simulink library "controlLibrary"  (R2019b)
settings: Solver=VariableStepAuto  StartTime=0.0  StopTime=10.0  RelTol=1e-3
undefined symbols (not defined in the file or in its folder): DiscIntNeverNeededParam, Up
libraries: simulink x5
settings Model: Creator=mwalker  LastModifiedBy=agonzale

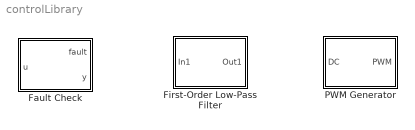
== system controlLibrary ==
  Fault Check : MATLAB Function  TreatAsAtomicUnit=on
  First-Order Low-Pass Filter : Subsystem  mask(First-Order Low-Pass Filter){fc=0.1}
      mask prompts: fc "Filter Constant"
      mask Display: disp(get_param(gcb,'fc'))
  PWM Generator : Subsystem  mask(PWM Generator){CarrCount=Up, Tper=0.001/0.05, Ts=0.001}
      mask prompts: CarrCount "Carrier counter:"; Tper "Timer period (s):"; Ts "Sample time"
      mask help:
      | This block implements a PWM generator.
      |
      | For discrete-time, set Sample time to a positive value. For continuous-time, set Sample time to zero.
      mask TypeOptions CarrCount: Carrier counter/CarrCount
      mask TypeOptions Tper: Carrier counter/Tper
      mask TypeOptions Ts: Carrier counter/Ts

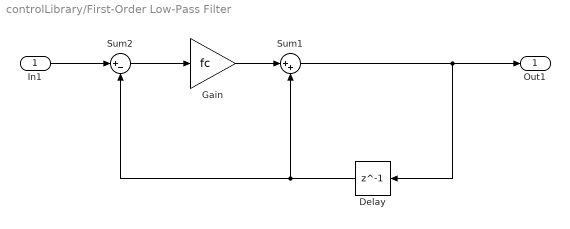
== system controlLibrary/First-Order Low-Pass Filter ==
  In1 : Inport
  Delay : Delay  DelayLength=1  InitialCondition=0
  Gain : Gain  Gain=fc
  Sum1 : Sum  Inputs=|++
  Sum2 : Sum  Inputs=|+-
  Out1 : Outport
  wires:
  In1/1 -> Sum2/1
  Sum1/1 -> Out1/1, Delay/1
  Sum2/1 -> Gain/1
  Delay/1 -> Sum2/2, Sum1/2
  Gain/1 -> Sum1/1

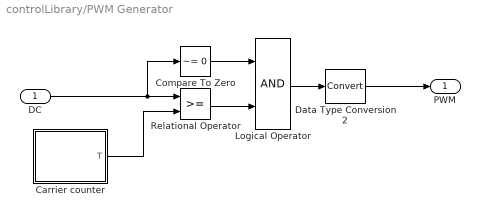
== system controlLibrary/PWM Generator ==
  DC : Inport  SampleTime=Ts
  Carrier counter : Subsystem  mask(Counter){CarrCount=Up, Range=[0 1], Tper=Tper, Tdelay=0, Ts=Ts}
      mask prompts: CarrCount "Counter type"; Range "Output range"; Tper "Timer period (s)"; Tdelay "Phase delay (s)"; Ts "Sample time"
      mask help:
      | This block implements a counter in either discrete or continuous time.
      |
      | For discrete-time, set Sample time to a positive value. For continuous-time, set Sample time to zero.
      mask init:
      | if CarrCount < 2.5
      |     Tdelay = mod(Tdelay,Tper);
      | else
      |     Tdelay = mod(Tdelay,2*Tper);
      | end
      | 
      | timeDomain = 'Discrete';
      mask TypeOptions CarrCount: physmod:ee:library:comments:control:eeGeneralControl:Up_PV | physmod:ee:library:comments:control:eeGeneralControl:Down_PV | physmod:ee:library:comments:control:eeGeneralControl:Up0x2DDown_PV
      mask TypeOptions Range: physmod:ee:library:comments:control:eeGeneralControl:x01_PV | physmod:ee:library:comments:control:eeGeneralControl:x0x2D11_PV
      mask TypeOptions Ts:
      | Integrator with
      | Wrapped State
      | (Discrete or Continuous)/Ts | Integrator with
      | Wrapped State
      | (Discrete or Continuous)1/Ts
      mask DialogControl ParameterGroupVar Prompt: physmod:ee:library:comments:control:eeGeneralControl:tab_Parameters
  Compare To Zero : simulink/Logic and Bit Operations/Compare To Zero  relop=~=  OutDataTypeStr=boolean
  Data Type Conversion2 : DataTypeConversion
  Logical Operator : Logic  AllPortsSameDT=off  OutDataTypeStr=boolean
  Relational Operator : RelationalOperator  OutDataTypeStr=boolean  RndMeth=Simplest
  PWM : Outport  VectorParamsAs1DForOutWhenUnconnected=off
  wires:
  Carrier counter/1(T) -> Relational Operator/2
  Logical Operator/1 -> Data Type Conversion2/1
  Compare To Zero/1 -> Logical Operator/1
  Relational Operator/1 -> Logical Operator/2
  DC/1 -> Compare To Zero/1, Relational Operator/1
  Data Type Conversion2/1 -> PWM/1

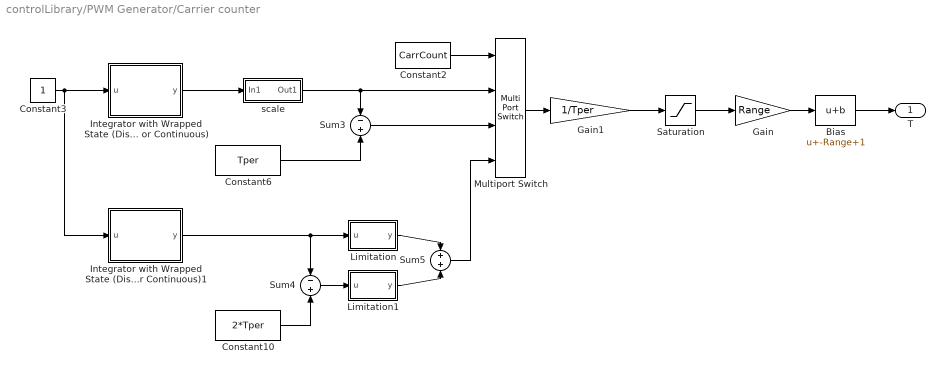
== system controlLibrary/PWM Generator/Carrier counter ==
  Bias : Bias  Bias=-Range+1
  Constant10 : Constant  Value=2*Tper  SampleTime=Ts
  Constant2 : Constant  Value=CarrCount  SampleTime=Ts
  Constant3 : Constant  SampleTime=Ts
  Constant6 : Constant  Value=Tper  SampleTime=Ts
  Gain : Gain  Gain=Range
  Gain1 : Gain  Gain=1/Tper
  Integrator with Wrapped State (Discrete or Continuous) : Subsystem  VariantControlMode=Label  Variant=on  LabelModeActiveChoice=Discrete  mask(Integrator with Wrapped State (Discrete or Continuous)){WrappedStateUpperValue=Tper, WrappedStateLowerValue=0, x0=Tdelay, Ts=Ts}
      mask prompts: WrappedStateUpperValue "Wrapped state upper value"; WrappedStateLowerValue "Wrapped state lower value"; x0 "Initial condition"; Ts "Sample time (-1 for inherited)"
      mask help:
      | This block models a discrete-time or continuous-time integrator with a wrapped state.
      |
      | For inherited discrete-time, set Sample time to -1. For discrete-time, set Sample time to a positive value. For continuous-time, set Sample time to zero.
      |
      | Use this block to represent a Voltage Controlled Oscillator (VCO).
      mask init:
      | timeDomain = 'Discrete';
      mask DialogControl ParameterGroupVar Prompt: physmod:ee:library:comments:control:eeGeneralControl:tab_Parameters
  Integrator with Wrapped State (Discrete or Continuous)1 : Subsystem  VariantControlMode=Label  Variant=on  LabelModeActiveChoice=Discrete  mask(Integrator with Wrapped State (Discrete or Continuous)){WrappedStateUpperValue=2*Tper, WrappedStateLowerValue=0, x0=Tdelay, Ts=Ts}
      mask prompts: WrappedStateUpperValue "Wrapped state upper value"; WrappedStateLowerValue "Wrapped state lower value"; x0 "Initial condition"; Ts "Sample time (-1 for inherited)"
      mask help:
      | This block models a discrete-time or continuous-time integrator with a wrapped state.
      |
      | For inherited discrete-time, set Sample time to -1. For discrete-time, set Sample time to a positive value. For continuous-time, set Sample time to zero.
      |
      | Use this block to represent a Voltage Controlled Oscillator (VCO).
      mask init:
      | timeDomain = 'Discrete';
      mask DialogControl ParameterGroupVar Prompt: physmod:ee:library:comments:control:eeGeneralControl:tab_Parameters
  Limitation : Subsystem
  Limitation1 : Subsystem
  Multiport Switch : MultiPortSwitch
  Saturation : Saturate  UpperLimit=1  LowerLimit=0
  Sum3 : Sum  Inputs=-+
  Sum4 : Sum  Inputs=-+
  Sum5 : Sum
  scale : Subsystem
  T : Outport  VectorParamsAs1DForOutWhenUnconnected=off
  wires:
  Integrator with Wrapped State (Discrete or Continuous)/1(y) -> scale/1(In1)
  Integrator with Wrapped State (Discrete or Continuous)1/1(y) -> Limitation/1(u), Sum4/1
  Multiport Switch/1 -> Gain1/1
  Constant3/1 -> Integrator with Wrapped State (Discrete or Continuous)1/1(u), Integrator with Wrapped State (Discrete or Continuous)/1(u)
  Sum3/1 -> Multiport Switch/3
  Constant10/1 -> Sum4/2
  Limitation/1(y) -> Sum5/1
  Sum5/1 -> Multiport Switch/4
  scale/1(Out1) -> Multiport Switch/2, Sum3/1
  Limitation1/1(y) -> Sum5/2
  Constant6/1 -> Sum3/2
  Sum4/1 -> Limitation1/1(u)
  Constant2/1 -> Multiport Switch/1
  Gain/1 -> Bias/1
  Gain1/1 -> Saturation/1
  Bias/1 -> T/1
  Saturation/1 -> Gain/1

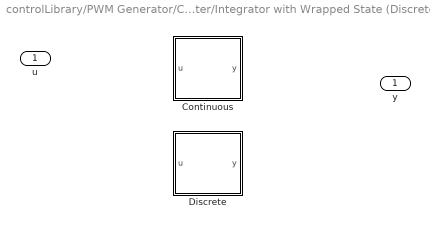
== system controlLibrary/PWM Generator/Carrier counter/Integrator with Wrapped State (Discrete or Continuous) ==
  u : Inport
  Continuous : Subsystem  VariantControl=Continuous
  Discrete : Subsystem  VariantControl=Discrete
  y : Outport  VectorParamsAs1DForOutWhenUnconnected=off

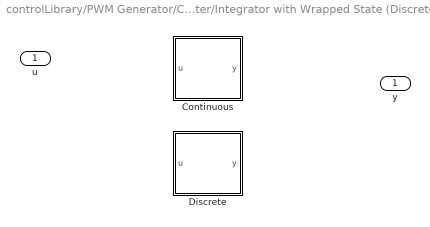
== system controlLibrary/PWM Generator/Carrier counter/Integrator with Wrapped State (Discrete or Continuous)1 ==
  u : Inport
  Continuous : Subsystem  VariantControl=Continuous
  Discrete : Subsystem  VariantControl=Discrete
  y : Outport  VectorParamsAs1DForOutWhenUnconnected=off

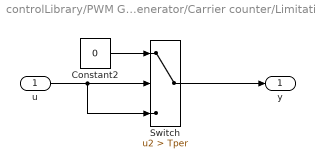
== system controlLibrary/PWM Generator/Carrier counter/Limitation ==
  u : Inport
  Constant2 : Constant  Value=0  SampleTime=Ts
  Switch : Switch  Criteria=u2 > Threshold  Threshold=Tper
  y : Outport  VectorParamsAs1DForOutWhenUnconnected=off
  wires:
  u/1 -> Switch/2, Switch/3
  Switch/1 -> y/1
  Constant2/1 -> Switch/1

== system controlLibrary/PWM Generator/Carrier counter/Limitation1 ==
  u : Inport
  Constant2 : Constant  Value=0  SampleTime=Ts
  Switch : Switch  Criteria=u2 > Threshold  Threshold=Tper
  y : Outport  VectorParamsAs1DForOutWhenUnconnected=off
  wires:
  Constant2/1 -> Switch/1
  Switch/1 -> y/1
  u/1 -> Switch/3, Switch/2

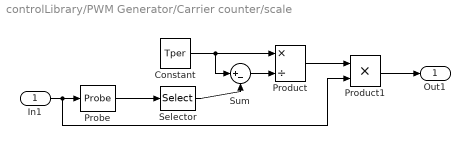
== system controlLibrary/PWM Generator/Carrier counter/scale ==
  In1 : Inport
  Constant : Constant  Value=Tper  SampleTime=Ts
  Probe : Probe  ProbeWidth=off  ProbeComplexSignal=off
  Product : Product  Inputs=*/
  Product1 : Product
  Selector : Selector  InputPortWidth=2  IndexOptions=Index vector (dialog)  Indices=1  OutputSizes=1
  Sum : Sum  Inputs=|+-
  Out1 : Outport  VectorParamsAs1DForOutWhenUnconnected=off
  wires:
  Probe/1 -> Selector/1
  In1/1 -> Product1/2, Probe/1
  Selector/1 -> Sum/2
  Constant/1 -> Sum/1, Product/1
  Sum/1 -> Product/2
  Product/1 -> Product1/1
  Product1/1 -> Out1/1

== system controlLibrary/PWM Generator/Carrier counter/Integrator with Wrapped State (Discrete or Continuous)/Continuous ==
  u : Inport
  Integrator : Integrator  InitialCondition=x0  WrapState=on  WrappedStateUpperValue=WrappedStateUpperValue  WrappedStateLowerValue=WrappedStateLowerValue
  y : Outport  VectorParamsAs1DForOutWhenUnconnected=off
  wires:
  u/1 -> Integrator/1
  Integrator/1 -> y/1

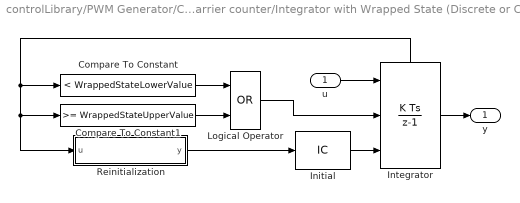
== system controlLibrary/PWM Generator/Carrier counter/Integrator with Wrapped State (Discrete or Continuous)/Discrete ==
  u : Inport
  Compare To Constant : simulink/Logic and Bit Operations/Compare To Constant  relop=<  const=WrappedStateLowerValue  OutDataTypeStr=boolean
  Compare To Constant1 : simulink/Logic and Bit Operations/Compare To Constant  relop=>=  const=WrappedStateUpperValue  OutDataTypeStr=boolean
  Initial : InitialCondition  Value=x0
  Integrator : DiscreteIntegrator  ExternalReset=rising  InitialConditionSource=external  SampleTime=Ts  ShowStatePort=on  ICPrevOutput=DiscIntNeverNeededParam  ICPrevScaledInput=DiscIntNeverNeededParam
  Logical Operator : Logic  Operator=OR  AllPortsSameDT=off  OutDataTypeStr=boolean
  Reinitialization : Subsystem
  y : Outport  VectorParamsAs1DForOutWhenUnconnected=off
  wires:
  Reinitialization/1(y) -> Initial/1
  Compare To Constant/1 -> Logical Operator/1
  Integrator/1 -> y/1
  Integrator/State -> Compare To Constant1/1, Reinitialization/1(u), Compare To Constant/1
  Compare To Constant1/1 -> Logical Operator/2
  Initial/1 -> Integrator/3
  u/1 -> Integrator/1
  Logical Operator/1 -> Integrator/2

== system controlLibrary/PWM Generator/Carrier counter/Integrator with Wrapped State (Discrete or Continuous)1/Continuous ==
  u : Inport
  Integrator : Integrator  InitialCondition=x0  WrapState=on  WrappedStateUpperValue=WrappedStateUpperValue  WrappedStateLowerValue=WrappedStateLowerValue
  y : Outport  VectorParamsAs1DForOutWhenUnconnected=off
  wires:
  u/1 -> Integrator/1
  Integrator/1 -> y/1

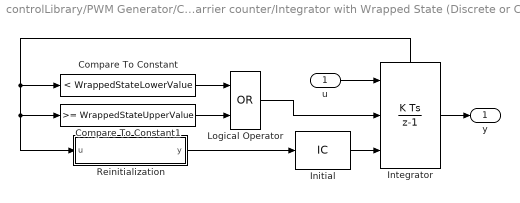
== system controlLibrary/PWM Generator/Carrier counter/Integrator with Wrapped State (Discrete or Continuous)1/Discrete ==
  u : Inport
  Compare To Constant : simulink/Logic and Bit Operations/Compare To Constant  relop=<  const=WrappedStateLowerValue  OutDataTypeStr=boolean
  Compare To Constant1 : simulink/Logic and Bit Operations/Compare To Constant  relop=>=  const=WrappedStateUpperValue  OutDataTypeStr=boolean
  Initial : InitialCondition  Value=x0
  Integrator : DiscreteIntegrator  ExternalReset=rising  InitialConditionSource=external  SampleTime=Ts  ShowStatePort=on  ICPrevOutput=DiscIntNeverNeededParam  ICPrevScaledInput=DiscIntNeverNeededParam
  Logical Operator : Logic  Operator=OR  AllPortsSameDT=off  OutDataTypeStr=boolean
  Reinitialization : Subsystem
  y : Outport  VectorParamsAs1DForOutWhenUnconnected=off
  wires:
  Reinitialization/1(y) -> Initial/1
  Compare To Constant/1 -> Logical Operator/1
  Integrator/1 -> y/1
  Integrator/State -> Compare To Constant1/1, Reinitialization/1(u), Compare To Constant/1
  Compare To Constant1/1 -> Logical Operator/2
  Initial/1 -> Integrator/3
  u/1 -> Integrator/1
  Logical Operator/1 -> Integrator/2

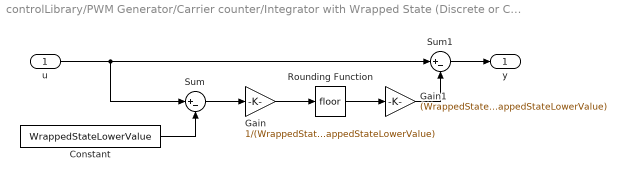
== system controlLibrary/PWM Generator/Carrier counter/Integrator with Wrapped State (Discrete or Continuous)/Discrete/Reinitialization ==
  u : Inport
  Constant : Constant  Value=WrappedStateLowerValue
  Gain : Gain  Gain=1/(WrappedStateUpperValue-WrappedStateLowerValue)
  Gain1 : Gain  Gain=(WrappedStateUpperValue-WrappedStateLowerValue)
  Rounding Function : Rounding
  Sum : Sum  Inputs=|+-
  Sum1 : Sum  Inputs=|+-
  y : Outport  VectorParamsAs1DForOutWhenUnconnected=off
  wires:
  Sum1/1 -> y/1
  Rounding Function/1 -> Gain1/1
  Constant/1 -> Sum/2
  Sum/1 -> Gain/1
  u/1 -> Sum1/1, Sum/1
  Gain/1 -> Rounding Function/1
  Gain1/1 -> Sum1/2

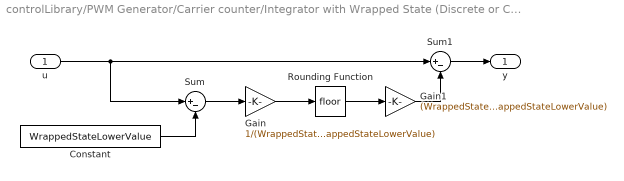
== system controlLibrary/PWM Generator/Carrier counter/Integrator with Wrapped State (Discrete or Continuous)1/Discrete/Reinitialization ==
  u : Inport
  Constant : Constant  Value=WrappedStateLowerValue
  Gain : Gain  Gain=1/(WrappedStateUpperValue-WrappedStateLowerValue)
  Gain1 : Gain  Gain=(WrappedStateUpperValue-WrappedStateLowerValue)
  Rounding Function : Rounding
  Sum : Sum  Inputs=|+-
  Sum1 : Sum  Inputs=|+-
  y : Outport  VectorParamsAs1DForOutWhenUnconnected=off
  wires:
  Sum1/1 -> y/1
  Rounding Function/1 -> Gain1/1
  Constant/1 -> Sum/2
  Sum/1 -> Gain/1
  u/1 -> Sum1/1, Sum/1
  Gain/1 -> Rounding Function/1
  Gain1/1 -> Sum1/2

== matlab function controlLibrary/Fault Check ==
  data: u input; fault output; y output
function [fault,y] = faultCheck(u)

if u > single(4.5) || u < single(0.5)
    fault = true;
    y = single(2.5); % Choose an appropriate default value
else
    fault = false;
    y = u; % Pass the input through
end
